simulink model "LKAS_AutoSave_20200910_1510"  (R2018b)
settings: Solver=FixedStepDiscrete  StartTime=0.0  StopTime=10.0  FixedStep=0.01  RelTol=1e-3
InitFcn:
  | tmpVer = ver('MATLAB');
  | tmpVer = str2num(tmpVer.Version);
  | % -------------------------------------------------------------------
  | %  MATLAB file generated by Simulink.saveVars on 21-Nov-2019 10:06:14
  | %  MATLAB version: 7.13.0.564 (R2011b)
  | % -------------------------------------------------------------------
  | 
  | 
  | SInt16 = Simulink.AliasType;
  | SInt16.Description = 'Num';
  | if (tmpVer > 7.11)
  | 	SInt16.DataScope = 'Auto';
  | end
  | SInt16.HeaderFile = 'Rte_Type.h';
  | SInt16.BaseType = 'int16';
  | 
  | SInt32 = Simulink.AliasType;
  | SInt32.Description = 'Num';
  | if (tmpVer > 7.11)
  | 	SInt32.DataScope = 'Auto';
  | end
  | SInt32.HeaderFile = 'Rte_Type.h';
  | SInt32.BaseType = 'int32';
  | 
  | SInt8 = Simulink.AliasType;
  | SInt8.Description = 'Num';
  | if (tmpVer > 7.11)
  | 	SInt8.DataScope = 'Auto';
  | end
  | SInt8.HeaderFile = 'Rte_Type.h';
  | SInt8.BaseType = 'int8';
  | 
  | T_A_m2_1024_1_u32 = Simulink.NumericType;
  | T_A_m2_1024_1_u32.Description = 'm2 (square meters  (m2))';
  | if (tmpVer > 7.11)
  | 	T_A_m2_1024_1_u32.DataScope = 'Auto';
  | end
  | T_A_m2_1024_1_u32.HeaderFile = 'Rte_Type.h';
  | T_A_m2_1024_1_u32.DataTypeMode = 'Fixed-point: slope and bias scaling';
  | T_A_m2_1024_1_u32.SignednessBool = false;
  | T_A_m2_1024_1_u32.WordLength = 32;
  | T_A_m2_1024_1_u32.FixedExponent = -10;
  | T_A_m2_1024_1_u32.SlopeAdjustmentFactor = 1;
  | T_A_m2_1024_1_u32.Bias = 0;
  | T_A_m2_1024_1_u32.DataTypeOverride = 'Inherit';
  | T_A_m2_1024_1_u32.IsAlias = true;
  | 
  | T_A_m2_65536_1_u16 = Simulink.NumericType;
  | T_A_m2_65536_1_u16.Description = 'm2 (square meters  (m2))';
  | if (tmpVer > 7.11)
  | 	T_A_m2_65536_1_u16.DataScope = 'Auto';
  | end
  | T_A_m2_65536_1_u16.HeaderFile = 'Rte_Type.h';
  | T_A_m2_65536_1_u16.DataTypeMode = 'Fixed-point: slope and bias scaling';
  | T_A_m2_65536_1_u16.SignednessBool = false;
  | T_A_m2_65536_1_u16.WordLength = 16;
  | T_A_m2_65536_1_u16.FixedExponent = -16;
  | T_A_m2_65536_1_u16.SlopeAdjustmentFactor = 1;
  | T_A_m2_65536_1_u16.Bias = 0;
  | T_A_m2_65536_1_u16.DataTypeOverride = 'Inherit';
  | ... (+4598 lines)
StopFcn:
  | clear  T_A_m2_1024_1_u32 T_A_m2_65536_1_u16 T_A_m2_Float32 T_A_mm2_10_1_u16 T_A_mm2_4_1_s16 T_A_mm2_Float32 T_Cnt_Num_10_1_u32 T_Cnt_Num_1_1_s16 T_Cnt_Num_1_1_s32 T_Cnt_Num_1_1_s8 T_Cnt_Num_1_1_u16 T_Cnt_Num_1_1_u32 T_Cnt_Num_1_1_u8 T_E_J_1_1_s32 T_E_J_Float32 T_E_kJ_128_1_s32 T_E_kJ_Float32 T_E_kwh_10_1_u16 T_E_kwh_Float32 T_Epl_kwhpkm_100_1_u16 T_Epl_kwhpkm_Float32 T_F_N_1_1_s16 T_F_N_Float32 T_I_A_1000_1_u16 T_I_A_1048576_1_s32 T_I_A_2048_1_s16 T_I_A_32_1_s16 T_I_A_Float32 T_I_mA_1_1_s16 T_I_mA_32768_128_s16 T_I_mA_Float32 T_J_kgpm2_128_1_u16 T_J_kgpm2_Float32 T_K_NA_1000_1_s16 T_K_NA_100_1_s16 T_K_NA_100_1_u16 T_K_NA_1024_1_s16 T_K_NA_1024_1_u16 T_K_NA_128_1_s16 T_K_NA_128_1_u16 T_K_NA_128_1_u8 T_K_NA_16777216_1_u32 T_K_NA_16_1_s16 T_K_NA_16_1_u16 T_K_NA_16_1_u8 T_K_NA_1_16_u16 T_K_NA_1_1_s16 T_K_NA_1_1_u16 T_K_NA_1_1_u8 T_K_NA_32768_1_s16 T_K_NA_32768_1_u16 T_K_NA_32_1_s8 T_K_NA_4096_1_u16 T_K_NA_4194304_1_s32 T_K_NA_4194304_1_u16 T_K_NA_65536_1_s32 T_K_NA_65536_1_u16 T_K_NA_8192_1_s16 T_K_NA_8_1_s16 T_K_NA_Float32 T_M_Nm_16_1_s16 T_M_Nm_1_1_s16 T_M_Nm_32768_1_s16 T_M_Nm_32_1_s16 T_M_Nm_4_1_s16 T_M_Nm_512_1_s16 T_M_Nm_Float32 T_P_W_1_4_s16 T_P_W_1_8_s16 T_P_W_Float32 T_P_kW_128_1_s16 T_P_kW_1_8_s16 T_P_kW_8_1_s32 T_P_kW_Float32 T_Pct_pct_1024_1_s32 T_Pct_pct_1024_1_u32 T_Pct_pct_10_1_s16 T_Pct_pct_10_1_u32 T_Pct_pct_128_100_s8 T_Pct_pct_1_1_s16 T_Pct_pct_1_4_u8 T_Pct_pct_255_100_u16 T_Pct_pct_255_100_u8 T_Pct_pct_256_1_s16 T_Pct_pct_256_1_u16 T_Pct_pct_65535_100_u16 T_Pct_pct_Float32 T_R_ohm_1024_1_s16 T_R_ohm_32_1_s16 T_R_ohm_Float32 T_TK_K_16_1_s16 T_TK_K_Float32 T_T_degC_10_400_1_u16 T_T_degC_16_1_s16 T_T_degC_1_40_1_u8 T_T_degC_2_80_1_u8 T_T_degC_Float32 T_U_V_1000_1_u16 T_U_V_10_1_u8 T_U_V_200_1_u8 T_U_V_32_1_s16 T_U_V_4096_1_s16 T_U_V_512_1_s16 T_U_V_65535_8_u16 T_U_V_8192_1_u16 T_U_V_Float32 T_U_mV_1_1_s16 T_U_mV_256_20_u16 T_U_mV_Float32 T_V_l_256_1_s16 T_V_l_4096_1_s16 T_V_l_64_1_s16 T_V_l_65535_100_u16 T_V_l_Float32 T_V_ml_128_1_s16 T_V_ml_1_1_s16 T_V_ml_32768_1_s16 T_V_ml_Float32 T_V_ul_32_1_u16 T_V_ul_Float32 T_Vpl_clpkm_512_1_u16 T_Vpl_clpkm_Float32 T_a_kphps_16_1_s16 T_a_kphps_Float32 T_a_mps2_128_1_s16 T_a_mps2_Float32 T_c_MJpkg_256_1_s16 T_c_MJpkg_Float32 T_c_kJpgpK_1024_1_s16 T_c_kJpgpK_Float32 T_c_kJpkgpK_128_1_u16 T_c_kJpkgpK_Float32 T_chrg_Ah_1_1_s16 T_chrg_Ah_1_1_u16 T_chrg_Ah_1_1_u8 T_chrg_Ah_256_1_u16 T_chrg_Ah_4194304_1_s32 T_chrg_Ah_512_1_u16 T_chrg_Ah_8_1_u16 T_chrg_Ah_Float32 T_cmp_NA_100_1_s16 T_cmp_NA_128_1_s16 T_cmp_NA_16_1_s16 T_cmp_NA_32768_1_u16 T_cmp_NA_Float32 T_d2n_rpmps2_4_1_s16 T_d2n_rpmps2_Float32 T_dPct_pctps_16_1_s16 T_dPct_pctps_256_1_s16 T_dPct_pctps_Float32 T_dT_degCps_128_1_s16 T_dT_degCps_Float32 T_dV_lph_1_1_s16 T_dV_lph_Float32 T_dV_lpm_128_1_s16 T_dV_lpm_32_1_s16 T_dV_lpm_Float32 T_dV_lps_1024_1_u16 T_dV_lps_4_1_u16 T_dV_lps_Float32 T_dV_mlps_1024_1_s16 T_dV_mlps_Float32 T_d_BitField16 T_dm_gps_128_1_s16 T_dm_gps_128_1_u16 T_dm_gps_256_1_u16 T_dm_gps_Float32 T_dm_mgps_1_1_s16 T_dm_mgps_Float32 T_dn_rpmps_1_1_s16 T_dn_rpmps_2_1_s16 T_dn_rpmps_Float32 T_dp_Paps_1_1_s16 T_dp_Paps_Float32 T_dp_kPaps_1_1_s16 T_dp_kPaps_8_1_s16 T_dp_kPaps_Float32 T_dphi_degps_128_1_s16 T_dphi_degps_8_1_s16 T_dphi_degps_Float32 T_dr_ps_256_1_s16 T_dr_ps_Float32 T_drho_mgplps_1_2_s16 T_drho_mgplps_Float32 T_e_NA_1_1_u8 T_f_Hz_1_1_u16 T_f_Hz_1_1_u32 T_f_Hz_64_1_u16 T_f_Hz_8_1_s16 T_f_Hz_Float32 T_g_BitField32 T_l_km_16_1_s16 T_l_km_1_1_u16 T_l_km_1_1_u32 T_l_km_Float32 T_l_m_1024_1_s16 T_l_m_16_1_s16 T_l_m_1_1_u32 T_l_m_Float32 T_l_mm_16_1_s16 T_l_mm_1_1_u16 T_l_mm_4096_1_s16 T_l_mm_4_1_u8 T_l_mm_64_1_s16 T_l_mm_Float32 T_m_g_1_1_s16 T_m_g_2048_1_s16 T_m_g_32_1_u16 T_m_g_Float32 T_m_kg_1024_1_s16 T_m_kg_1_1_s16 T_m_kg_1_1_u32 T_m_kg_Float32 T_m_mg_128_1_s16 T_m_mg_32_1_s16 T_m_mg_Float32 T_n_rpm_1_1_s16 T_n_rpm_1_25_u8 T_n_rpm_256_50_u16 T_n_rpm_2_25_u8 T_n_rpm_4_1_u16 T_n_rpm_Float32 T_p_MPa_64_1_s16 T_p_MPa_Float32 T_p_Pa_1_1_s16 T_p_Pa_Float32 T_p_kPa_1_10_u16 T_p_kPa_1_1_s16 T_p_kPa_1_1_u8 T_p_kPa_256_1_u16 T_p_kPa_32_1_u16 T_p_kPa_64_1_s16 T_p_kPa_Float32 T_phi_deg_100_1_s16 T_phi_deg_1024_1_s16 T_phi_deg_128_1_s16 T_phi_deg_1_1_u8 T_phi_deg_256_1_s16 T_phi_deg_2_1_s8 T_phi_deg_32_1_s16 T_phi_deg_512_6_s32 T_phi_deg_Float32 T_phi_rad_2048_1_s16 T_phi_rad_Float32 T_r_NA_1024_1_s16 T_r_NA_1024_1_u16 T_r_NA_16384_1_s16 T_r_NA_16_1_s16 T_r_NA_256_1_s8 T_r_NA_256_1_u16 T_r_NA_32768_1_u16 T_r_NA_32_1_u16 T_r_NA_4096_1_s16 T_r_NA_65535_2_u16 T_r_NA_8192_1_u16 T_r_NA_Float32 T_rho_gpl_8192_1_s16 T_rho_gpl_Float32 T_rho_kgpm3_16_1_s16 T_rho_kgpm3_Float32 T_rho_mgpl_1_1_s16 T_rho_mgpl_64_1_s16 T_rho_mgpl_Float32 T_t_hour_1_1_s16 T_t_hour_Float32 T_t_m_1_1_u16 T_t_m_Float32 T_t_ms_1_1_s16 T_t_ms_1_1_u16 T_t_ms_1_1_u32 T_t_ms_4096_1_s16 T_t_ms_64_1_s16 T_t_ms_Float32 T_t_s_1000_1_s16 T_t_s_100_1_s16 T_t_s_10_1_s16 T_t_s_10_1_u16 T_t_s_1_1_s16 T_t_s_1_1_u16 T_t_s_1_1_u32 T_t_s_Float32 T_t_us_10_1_u32 T_t_us_1_1_s16 T_t_us_1_1_u32 T_t_us_1_4_u16 T_t_us_Float32 T_v_kph_1_1_u8 T_v_kph_64_1_s16 T_v_kph_64_1_u16 T_v_kph_Float32 T_v_mps_256_1_s16 T_v_mps_Float32 T_w_radps_32_1_s16 T_w_radps_Float32 T_y_BitField8 T_y_BitFieldDiagProgress T_y_BitFieldDiagStatus T_y_NA_1_1_u8 SInt16 SInt32 SInt8 T_BOOLEAN UInt16 UInt32 UInt8 s16 s32 s8 u16 u32 u8
model workspace (MAT data in the model file):
  MCOS : class17 (value not decoded)
  MCOS : class17 (value not decoded)
  MCOS : class17 (value not decoded)
  MCOS : class17 (value not decoded)
  MCOS : class17 (value not decoded)
  MCOS : class17 (value not decoded)
  MCOS : class17 (value not decoded)
  MCOS : class17 (value not decoded)
  MCOS : class17 (value not decoded)
  MCOS : class17 (value not decoded)
  MCOS : class17 (value not decoded)
  MCOS : class17 (value not decoded)
  MCOS : class17 (value not decoded)
  MCOS : class17 (value not decoded)
  MCOS : class17 (value not decoded)
  MCOS : class17 (value not decoded)
  MCOS : class17 (value not decoded)
  MCOS : class17 (value not decoded)
  MCOS : class17 (value not decoded)
  MCOS : class17 (value not decoded)
  MCOS : class17 (value not decoded)
  MCOS : class17 (value not decoded)
  MCOS : class17 (value not decoded)
  MCOS : class17 (value not decoded)
  MCOS : class17 (value not decoded)
  MCOS : class17 (value not decoded)
  MCOS : class17 (value not decoded)
  MCOS : class17 (value not decoded)
  MCOS : class17 (value not decoded)
  MCOS : class17 (value not decoded)
  MCOS : class17 (value not decoded)
  MCOS : class17 (value not decoded)
  MCOS : class17 (value not decoded)
  MCOS : class17 (value not decoded)
  MCOS : class17 (value not decoded)
  MCOS : class17 (value not decoded)
  MCOS : class17 (value not decoded)
  MCOS : class17 (value not decoded)
  MCOS : class17 (value not decoded)
  MCOS : class17 (value not decoded)
  MCOS : class17 (value not decoded)
  MCOS : class17 (value not decoded)
  MCOS : class17 (value not decoded)
  MCOS : class17 (value not decoded)
  MCOS : class17 (value not decoded)
  MCOS : class17 (value not decoded)
  MCOS : class17 (value not decoded)
  MCOS : class17 (value not decoded)
  MCOS : class17 (value not decoded)
  MCOS : class17 (value not decoded)
  MCOS : class17 (value not decoded)
  MCOS : class17 (value not decoded)
  MCOS : class17 (value not decoded)
  MCOS : class17 (value not decoded)
  MCOS : class17 (value not decoded)
  MCOS : class17 (value not decoded)
  MCOS : class17 (value not decoded)
  MCOS : class17 (value not decoded)
  MCOS : class17 (value not decoded)
  MCOS : class17 (value not decoded)
  MCOS : class17 (value not decoded)
  MCOS : class17 (value not decoded)
  MCOS : class17 (value not decoded)
  MCOS : class17 (value not decoded)
  MCOS : class17 (value not decoded)
  MCOS : class17 (value not decoded)
  MCOS : class17 (value not decoded)
  MCOS : class17 (value not decoded)
  MCOS : class17 (value not decoded)
  MCOS : class17 (value not decoded)
  MCOS : class17 (value not decoded)
  MCOS : class17 (value not decoded)
  MCOS : class17 (value not decoded)
  MCOS : class17 (value not decoded)
  MCOS : class17 (value not decoded)
  MCOS : class17 (value not decoded)
  MCOS : class17 (value not decoded)
  MCOS : class17 (value not decoded)
  MCOS : class17 (value not decoded)
  MCOS : class17 (value not decoded)
  MCOS : class17 (value not decoded)
  MCOS : class17 (value not decoded)
  MCOS : class17 (value not decoded)
  MCOS : class17 (value not decoded)
  MCOS : class17 (value not decoded)
  MCOS : class17 (value not decoded)
  MCOS : class17 (value not decoded)
  MCOS : class17 (value not decoded)
  MCOS : class17 (value not decoded)
undefined symbols (not defined in the file): LKA_CarWidth, LKA_SampleTime, LKA_StrRatio_C, LKA_Veh2CamL_C, LKA_Veh2CamW_C, LKA_WhlBaseL_C, LL_CompSWA_C, LL_CrvtPrvwT_C, LL_DesDvt_C, LL_DvtComp_C, LL_DvtPrvwT_C, LL_DvtSpdDet_vDvtSpdMin_C, LL_HdAgExT_C, LL_HdAgPrvwT_C, LL_LAccMax_C, LL_LAccRMax_C, LL_LDW_EarliestWarnLine_C, LL_LDW_LatestWarnLine_C, LL_LDWS_SUPPRESS_HEADING, LL_LFClb_TFC_DiffCtlBalance, LL_LFClb_TFC_DiffCtrlMaxSWA, LL_LFClb_TFC_DiffCtrlRatio, LL_LFClb_TFC_facmGainLutGain1_C, LL_LFClb_TFC_facmGainLutGain2_C, LL_LFClb_TFC_facmIntegRatio, LL_LFClb_TFC_facmKlat_C, LL_LFClb_TFC_FfCtlRatio_C, LL_LFClb_TFC_phiIntegCtlMaxSWA_C, LL_LFClb_TFC_tiKlatPrvwT_C, LL_LFClb_TFC_vGainLutVehSpdLwr_C, LL_LFClb_TFC_vGainLutVehSpdUpr_C, LL_LKA_EarliestWarnLine_C, LL_LKA_LatestWarnLine_C, LL_LKAExPrcs_ExitC0Dvt, LL_LKAExPrcs_ExitC0Swt, LL_LKAExPrcs_tiExitTime1, LL_LKAExPrcs_tiExitTime2, LL_LKAExPrcs_tiExitTime3, LL_LKAS_OUT_OF_CONTROL_LAT_VEL, LL_LKAS_OUT_OF_CONTROL_TTLC, LL_LKASWASyn_M0, LL_LKASWASyn_M1, LL_LKASWASyn_M2, LL_LKASWASyn_M3K, LL_LKASWASyn_SWAaddMax, LL_LKASWASyn_T2, LL_LKASWASyn_tiTrqSwaRtTime, LL_LKASWASyn_tiTrqSwaTime, LL_LKASWASyn_TrqMax, LL_LKASWASyn_TrqSwaAddSwt, LL_LKASWASyn_TrqSwaRateDiff, LL_LSpdCompT_C, LL_lStpLngth_C, LL_MAX_DELAY_EPSSTAR_TIME, LL_MAX_DRIVER_TORQUE_DISABLE, LL_MAX_DRIVER_TORQUE_ENABLE, LL_MAX_LANE_WIDTH_DISABLE, LL_MAX_LANE_WIDTH_ENABLE, LL_MAX_LAT_ACC_DISABLE, LL_MAX_LAT_ACC_ENABLE ... (+29)
libraries: simulink x134, dspstat3 x3, simulink_extras x1
(part 5 of 19)

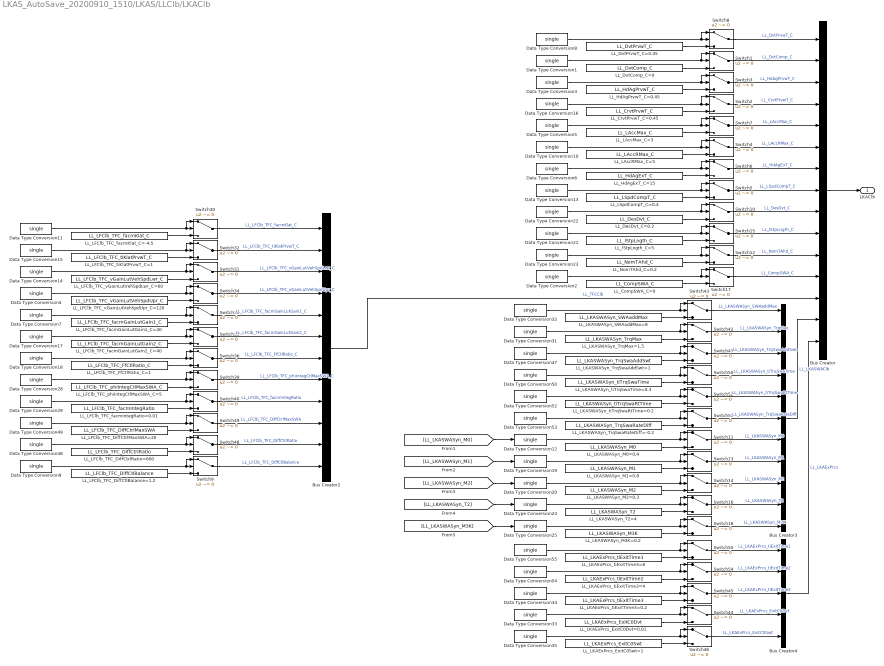
== system LKAS_AutoSave_20200910_1510/LKAS/LLClb/LKAClb ==
  Bus Creator : BusCreator  Inputs=15
  Bus Creator2 : BusCreator  Inputs=12
  Bus Creator3 : BusCreator  Inputs=11
  Bus Creator4 : BusCreator  Inputs=5
  Data Type Conversion{1..25,28..29,31..35,47..50,52..55} (40 alike) : DataTypeConversion  OutDataTypeStr=single
  LL_CompSWA_C=0 : Constant  Value=LL_CompSWA_C  OutDataTypeStr=single
  LL_CrvtPrvwT_C=0.45 : Constant  Value=LL_CrvtPrvwT_C  OutDataTypeStr=single
  LL_DesDvt_C=0.2 : Constant  Value=LL_DesDvt_C  OutDataTypeStr=single
  LL_DvtComp_C=0 : Constant  Value=LL_DvtComp_C  OutDataTypeStr=single
  LL_DvtPrvwT_C=0.45 : Constant  Value=LL_DvtPrvwT_C  OutDataTypeStr=single
  LL_HdAgExT_C=15 : Constant  Value=LL_HdAgExT_C  OutDataTypeStr=single
  LL_HdAgPrvwT_C=0.45 : Constant  Value=LL_HdAgPrvwT_C  OutDataTypeStr=single
  LL_LAccMax_C=3 : Constant  Value=LL_LAccMax_C  OutDataTypeStr=single
  LL_LAccRMax_C=5 : Constant  Value=LL_LAccRMax_C  OutDataTypeStr=single
  LL_LFClb_TFC_DiffCtlBalance=1.2 : Constant  Value=LL_LFClb_TFC_DiffCtlBalance  OutDataTypeStr=single
  LL_LFClb_TFC_DiffCtrlMaxSWA=20 : Constant  Value=LL_LFClb_TFC_DiffCtrlMaxSWA  OutDataTypeStr=single
  LL_LFClb_TFC_DiffCtrlRatio=600 : Constant  Value=LL_LFClb_TFC_DiffCtrlRatio  OutDataTypeStr=single
  LL_LFClb_TFC_FfCtlRatio_C=1 : Constant  Value=LL_LFClb_TFC_FfCtlRatio_C  OutDataTypeStr=single
  LL_LFClb_TFC_facmGainLutGain1_C=40 : Constant  Value=LL_LFClb_TFC_facmGainLutGain1_C  OutDataTypeStr=single
  LL_LFClb_TFC_facmGainLutGain2_C=40 : Constant  Value=LL_LFClb_TFC_facmGainLutGain2_C  OutDataTypeStr=single
  LL_LFClb_TFC_facmIntegRatio=0.01 : Constant  Value=LL_LFClb_TFC_facmIntegRatio  OutDataTypeStr=single
  LL_LFClb_TFC_facmKlat_C=-4.5 : Constant  Value=LL_LFClb_TFC_facmKlat_C  OutDataTypeStr=single
  LL_LFClb_TFC_phiIntegCtlMaxSWA_C=5 : Constant  Value=LL_LFClb_TFC_phiIntegCtlMaxSWA_C  OutDataTypeStr=single
  LL_LFClb_TFC_tiKlatPrvwT_C=1 : Constant  Value=LL_LFClb_TFC_tiKlatPrvwT_C  OutDataTypeStr=single
  LL_LFClb_TFC_vGainLutVehSpdLwr_C=60 : Constant  Value=LL_LFClb_TFC_vGainLutVehSpdLwr_C  OutDataTypeStr=single
  LL_LFClb_TFC_vGainLutVehSpdUpr_C=120 : Constant  Value=LL_LFClb_TFC_vGainLutVehSpdUpr_C  OutDataTypeStr=single
  LL_LKAExPrcs_ExitC0Dvt=0.01 : Constant  Value=LL_LKAExPrcs_ExitC0Dvt  OutDataTypeStr=single
  LL_LKAExPrcs_ExitC0Swt=1 : Constant  Value=LL_LKAExPrcs_ExitC0Swt  OutDataTypeStr=single
  LL_LKAExPrcs_tiExitTime3=0.2 : Constant  Value=LL_LKAExPrcs_tiExitTime3  OutDataTypeStr=single
  LL_LKAExPrcs_tiExitTime3=4 : Constant  Value=LL_LKAExPrcs_tiExitTime2  OutDataTypeStr=single
  LL_LKAExPrcs_tiExitTime3=8 : Constant  Value=LL_LKAExPrcs_tiExitTime1  OutDataTypeStr=single
  LL_LKASWASyn_M0=0.4 : Constant  Value=LL_LKASWASyn_M0  OutDataTypeStr=single
  LL_LKASWASyn_M1=0.8 : Constant  Value=LL_LKASWASyn_M1  OutDataTypeStr=single
  LL_LKASWASyn_M2=0.3 : Constant  Value=LL_LKASWASyn_M2  OutDataTypeStr=single
  LL_LKASWASyn_M3K=0.2 : Constant  Value=LL_LKASWASyn_M3K  OutDataTypeStr=single
  LL_LKASWASyn_SWAaddMax=8 : Constant  Value=LL_LKASWASyn_SWAaddMax  OutDataTypeStr=single
  LL_LKASWASyn_T2=4 : Constant  Value=LL_LKASWASyn_T2  OutDataTypeStr=single
  LL_LKASWASyn_TrqMax=1.5 : Constant  Value=LL_LKASWASyn_TrqMax  OutDataTypeStr=single
  LL_LKASWASyn_TrqSwaAddSwt=1 : Constant  Value=LL_LKASWASyn_TrqSwaAddSwt  OutDataTypeStr=single
  LL_LKASWASyn_TrqSwaRateDiff=-0.2 : Constant  Value=LL_LKASWASyn_TrqSwaRateDiff  OutDataTypeStr=single
  LL_LKASWASyn_tiTrqSwaRtTime=0.2 : Constant  Value=LL_LKASWASyn_tiTrqSwaRtTime  OutDataTypeStr=single
  LL_LKASWASyn_tiTrqSwaTime=0.3 : Constant  Value=LL_LKASWASyn_tiTrqSwaTime  OutDataTypeStr=single
  LL_LSpdCompT_C=0.4 : Constant  Value=LL_LSpdCompT_C  OutDataTypeStr=single
  LL_NomTAhd_C=0.2 : Constant  Value=LL_NomTAhd_C  OutDataTypeStr=single
  LL_lStpLngth_C=5 : Constant  Value=LL_lStpLngth_C  OutDataTypeStr=single
  Switch{1..18,30..36,39..40,42..50,52..55} (40 alike) : Switch  Criteria=u2 ~= 0  OutDataTypeStr=single
  LKAClb : Outport
  wires:
  [LL_LKASWASyn_M3K] -> Data Type Conversion25/1
  Switch18/1 -> Bus Creator3/11  "LL_LKASWASyn_M3K"
  LL_LKASWASyn_M3K=0.2/1 -> Switch18/3
  Data Type Conversion25/1 -> Switch18/1, Switch18/2
  [LL_LKASWASyn_M0] -> Data Type Conversion12/1
  Switch11/1 -> Bus Creator3/7  "LL_LKASWASyn_M0"
  LL_LKASWASyn_M0=0.4/1 -> Switch11/3
  Data Type Conversion12/1 -> Switch11/1, Switch11/2
  Data Type Conversion19/1 -> Switch13/2, Switch13/1
  LL_LKASWASyn_M1=0.8/1 -> Switch13/3
  Switch13/1 -> Bus Creator3/8  "LL_LKASWASyn_M1"
  [LL_LKASWASyn_M1] -> Data Type Conversion19/1
  [LL_LKASWASyn_M2] -> Data Type Conversion20/1
  Switch14/1 -> Bus Creator3/9  "LL_LKASWASyn_M2"
  LL_LKASWASyn_M2=0.3/1 -> Switch14/3
  Data Type Conversion20/1 -> Switch14/1, Switch14/2
  Data Type Conversion24/1 -> Switch16/2, Switch16/1
  LL_LKASWASyn_T2=4/1 -> Switch16/3
  Switch16/1 -> Bus Creator3/10  "LL_LKASWASyn_T2"
  [LL_LKASWASyn_T2] -> Data Type Conversion24/1
  Data Type Conversion9/1 -> Switch9/2, Switch9/1
  LL_LFClb_TFC_DiffCtlBalance=1.2/1 -> Switch9/3
  Switch9/1 -> Bus Creator2/12  "LL_LFClb_TFC_DiffCtlBalance"
  LL_LKAExPrcs_tiExitTime3=8/1 -> Switch55/3
  Data Type Conversion55/1 -> Switch55/1, Switch55/2
  Switch55/1 -> Bus Creator4/1  "LL_LKAExPrcs_tiExitTime1"
  Switch54/1 -> Bus Creator4/2  "LL_LKAExPrcs_tiExitTime2"
  Data Type Conversion54/1 -> Switch54/2, Switch54/1
  LL_LKAExPrcs_tiExitTime3=4/1 -> Switch54/3
  Switch53/1 -> Bus Creator3/6  "LL_LKASWASyn_TrqSwaRateDiff"
  LL_LKASWASyn_TrqSwaRateDiff=-0.2/1 -> Switch53/3
  Data Type Conversion53/1 -> Switch53/1, Switch53/2
  Data Type Conversion52/1 -> Switch52/2, Switch52/1
  LL_LKASWASyn_tiTrqSwaRtTime=0.2/1 -> Switch52/3
  Switch52/1 -> Bus Creator3/5  "LL_LKASWASyn_tiTrqSwaRtTime"
  Switch50/1 -> Bus Creator3/4  "LL_LKASWASyn_tiTrqSwaTime"
  LL_LKASWASyn_tiTrqSwaTime=0.3/1 -> Switch50/3
  Data Type Conversion50/1 -> Switch50/1, Switch50/2
  Data Type Conversion49/1 -> Switch49/2, Switch49/1
  LL_LFClb_TFC_DiffCtrlMaxSWA=20/1 -> Switch49/3
  Switch49/1 -> Bus Creator2/10  "LL_LFClb_TFC_DiffCtrlMaxSWA"
  Switch48/1 -> Bus Creator2/11  "LL_LFClb_TFC_DiffCtrlRatio"
  LL_LFClb_TFC_DiffCtrlRatio=600/1 -> Switch48/3
  Data Type Conversion48/1 -> Switch48/1, Switch48/2
  Data Type Conversion47/1 -> Switch47/2, Switch47/1
  LL_LKASWASyn_TrqSwaAddSwt=1/1 -> Switch47/3
  Switch47/1 -> Bus Creator3/3  "LL_LKASWASyn_TrqSwaAddSwt"
  Switch46/1 -> Bus Creator4/5  "LL_LKAExPrcs_ExitC0Swt"
  LL_LKAExPrcs_ExitC0Swt=1/1 -> Switch46/3
  Data Type Conversion35/1 -> Switch46/1, Switch46/2
  Bus Creator4/1 -> Bus Creator/15  "LL_LKAExPrcs"
  Data Type Conversion33/1 -> Switch44/2, Switch44/1
  LL_LKAExPrcs_ExitC0Dvt=0.01/1 -> Switch44/3
  LL_LKAExPrcs_tiExitTime3=0.2/1 -> Switch45/3
  Data Type Conversion34/1 -> Switch45/1, Switch45/2
  Switch45/1 -> Bus Creator4/3  "LL_LKAExPrcs_tiExitTime3"
  Switch44/1 -> Bus Creator4/4  "LL_LKAExPrcs_ExitC0Dvt"
  Bus Creator3/1 -> Bus Creator/14  "LL_LKASWAClb"
  Switch42/1 -> Bus Creator3/2  "LL_LKASWASyn_TrqMax"
  Switch43/1 -> Bus Creator3/1  "LL_LKASWASyn_SWAaddMax"
  Data Type Conversion32/1 -> Switch43/2, Switch43/1
  LL_LKASWASyn_SWAaddMax=8/1 -> Switch43/3
  LL_LKASWASyn_TrqMax=1.5/1 -> Switch42/3
  Data Type Conversion31/1 -> Switch42/1, Switch42/2
  Data Type Conversion29/1 -> Switch40/2, Switch40/1
  LL_LFClb_TFC_facmIntegRatio=0.01/1 -> Switch40/3
  Data Type Conversion28/1 -> Switch39/2, Switch39/1
  LL_LFClb_TFC_phiIntegCtlMaxSWA_C=5/1 -> Switch39/3
  Switch39/1 -> Bus Creator2/8  "LL_LFClb_TFC_phiIntegCtlMaxSWA_C"
  Switch40/1 -> Bus Creator2/9  "LL_LFClb_TFC_facmIntegRatio"
  Switch36/1 -> Bus Creator2/7  "LL_LFClb_TFC_FfCtlRatio_C"
  Data Type Conversion18/1 -> Switch36/2, Switch36/1
  LL_LFClb_TFC_FfCtlRatio_C=1/1 -> Switch36/3
  LL_LFClb_TFC_facmKlat_C=-4.5/1 -> Switch30/3
  LL_LFClb_TFC_vGainLutVehSpdUpr_C=120/1 -> Switch34/3
  Data Type Conversion14/1 -> Switch31/1, Switch31/2
  LL_LFClb_TFC_facmGainLutGain2_C=40/1 -> Switch35/3
  Data Type Conversion17/1 -> Switch35/1, Switch35/2
  Data Type Conversion15/1 -> Switch32/1, Switch32/2
  Data Type Conversion4/1 -> Switch34/1, Switch34/2
  Data Type Conversion7/1 -> Switch33/1, Switch33/2
  Data Type Conversion11/1 -> Switch30/1, Switch30/2
  LL_LFClb_TFC_tiKlatPrvwT_C=1/1 -> Switch32/3
  LL_LFClb_TFC_vGainLutVehSpdLwr_C=60/1 -> Switch31/3
  LL_LFClb_TFC_facmGainLutGain1_C=40/1 -> Switch33/3
  Switch32/1 -> Bus Creator2/2  "LL_LFClb_TFC_tiKlatPrvwT_C"
  Switch33/1 -> Bus Creator2/5  "LL_LFClb_TFC_facmGainLutGain1_C"
  Switch34/1 -> Bus Creator2/4  "LL_LFClb_TFC_vGainLutVehSpdUpr_C"
  Switch31/1 -> Bus Creator2/3  "LL_LFClb_TFC_vGainLutVehSpdLwr_C"
  Switch30/1 -> Bus Creator2/1  "LL_LFClb_TFC_facmKlat_C"
  Switch35/1 -> Bus Creator2/6  "LL_LFClb_TFC_facmGainLutGain2_C"
  Bus Creator2/1 -> Bus Creator/13  "LL_TFCClb"
  LL_CompSWA_C=0/1 -> Switch17/3
  LL_NomTAhd_C=0.2/1 -> Switch12/3
  LL_lStpLngth_C=5/1 -> Switch15/3
  LL_DesDvt_C=0.2/1 -> Switch10/3
  Data Type Conversion2/1 -> Switch17/1, Switch17/2
  Data Type Conversion22/1 -> Switch10/1, Switch10/2
  Data Type Conversion23/1 -> Switch12/1, Switch12/2
  Data Type Conversion21/1 -> Switch15/1, Switch15/2
  LL_LAccMax_C=3/1 -> Switch7/3
  Data Type Conversion5/1 -> Switch7/1, Switch7/2
  Data Type Conversion10/1 -> Switch4/2, Switch4/1
  LL_LAccRMax_C=5/1 -> Switch4/3
  LL_LSpdCompT_C=0.4/1 -> Switch5/3
  Data Type Conversion13/1 -> Switch5/1, Switch5/2
  Data Type Conversion6/1 -> Switch6/1, Switch6/2
  LL_HdAgExT_C=15/1 -> Switch6/3
  LL_HdAgPrvwT_C=0.45/1 -> Switch3/3
  Data Type Conversion3/1 -> Switch3/1, Switch3/2
  Data Type Conversion16/1 -> Switch2/1, Switch2/2
  LL_CrvtPrvwT_C=0.45/1 -> Switch2/3
  LL_DvtComp_C=0/1 -> Switch1/3
  Data Type Conversion1/1 -> Switch1/1, Switch1/2
  Data Type Conversion8/1 -> Switch8/2, Switch8/1
  LL_DvtPrvwT_C=0.45/1 -> Switch8/3
  Switch12/1 -> Bus Creator/11  "LL_NomTAhd_C"
  Switch10/1 -> Bus Creator/9  "LL_DesDvt_C"
  Switch15/1 -> Bus Creator/10  "LL_lStpLngth_C"
  Switch2/1 -> Bus Creator/4  "LL_CrvtPrvwT_C"
  Switch5/1 -> Bus Creator/8  "LL_LSpdCompT_C"
  Switch4/1 -> Bus Creator/6  "LL_LAccRMax_C"
  Switch7/1 -> Bus Creator/5  "LL_LAccMax_C"
  Switch6/1 -> Bus Creator/7  "LL_HdAgExT_C"
  Switch17/1 -> Bus Creator/12  "LL_CompSWA_C"
  Switch3/1 -> Bus Creator/3  "LL_HdAgPrvwT_C"
  Switch1/1 -> Bus Creator/2  "LL_DvtComp_C"
  Switch8/1 -> Bus Creator/1  "LL_DvtPrvwT_C"
  Bus Creator/1 -> LKAClb/1

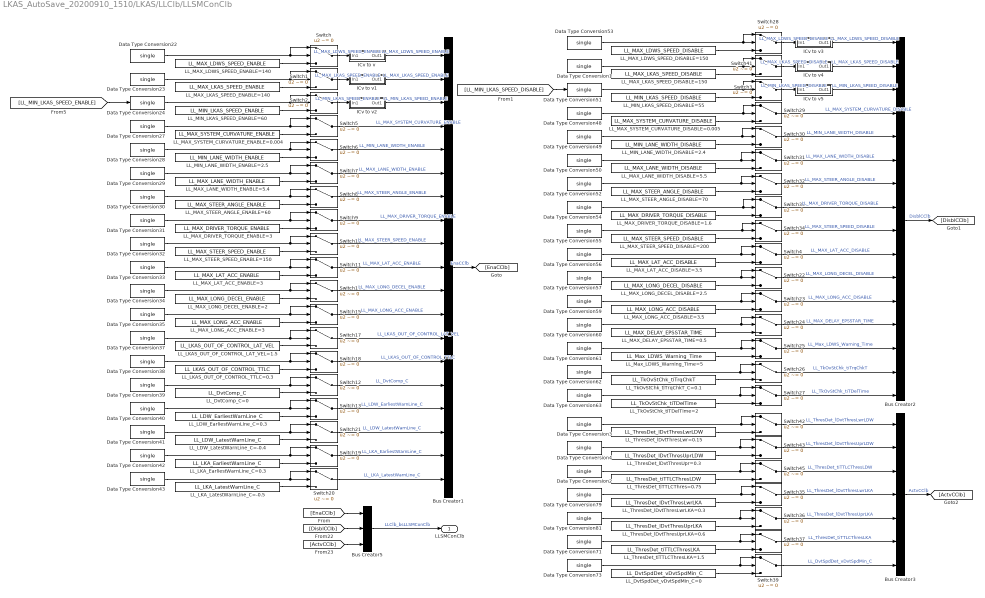
== system LKAS_AutoSave_20200910_1510/LKAS/LLClb/LLSMConClb ==
  Bus Creator1 : BusCreator  Inputs=19
  Bus Creator2 : BusCreator  Inputs=16
  Bus Creator3 : BusCreator  Inputs=7
  Bus Creator5 : BusCreator  Inputs=3
  Data Type Conversion{1..4,22..24,27..35,37..43,48..57,59..63,71,73,79,81} (42 alike) : DataTypeConversion  OutDataTypeStr=single
  ICv to v : Subsystem
  ICv to v1 : Subsystem
  ICv to v2 : Subsystem
  ICv to v3 : Subsystem
  ICv to v4 : Subsystem
  ICv to v5 : Subsystem
  LL_DvtComp_C=0 : Constant  Value=LL_DvtComp_C  OutDataTypeStr=single
  LL_DvtSpdDet_vDvtSpdMin_C=0 : Constant  Value=LL_DvtSpdDet_vDvtSpdMin_C  OutDataTypeStr=single
  LL_LDW_EarliestWarnLine_C=0.3 : Constant  Value=LL_LDW_EarliestWarnLine_C  OutDataTypeStr=single
  LL_LDW_LatestWarnLine_C=-0.4 : Constant  Value=LL_LDW_LatestWarnLine_C  OutDataTypeStr=single
  LL_LKAS_OUT_OF_CONTROL_LAT_VEL=1.5 : Constant  Value=LL_LKAS_OUT_OF_CONTROL_LAT_VEL  OutDataTypeStr=single
  LL_LKAS_OUT_OF_CONTROL_TTLC=0.3 : Constant  Value=LL_LKAS_OUT_OF_CONTROL_TTLC  OutDataTypeStr=single
  LL_LKA_EarliestWarnLine_C=0.3 : Constant  Value=LL_LKA_EarliestWarnLine_C  OutDataTypeStr=single
  LL_LKA_LatestWarnLine_C=-0.5 : Constant  Value=LL_LKA_LatestWarnLine_C  OutDataTypeStr=single
  LL_MAX_DELAY_EPSSTAR_TIME=0.5 : Constant  Value=LL_MAX_DELAY_EPSSTAR_TIME  OutDataTypeStr=single
  LL_MAX_DRIVER_TORQUE_DISABLE=1.6 : Constant  Value=LL_MAX_DRIVER_TORQUE_DISABLE  OutDataTypeStr=single
  LL_MAX_DRIVER_TORQUE_ENABLE=3 : Constant  Value=LL_MAX_DRIVER_TORQUE_ENABLE  OutDataTypeStr=single
  LL_MAX_LANE_WIDTH_DISABLE=5.5 : Constant  Value=LL_MAX_LANE_WIDTH_DISABLE  OutDataTypeStr=single
  LL_MAX_LANE_WIDTH_ENABLE=5.4 : Constant  Value=LL_MAX_LANE_WIDTH_ENABLE  OutDataTypeStr=single
  LL_MAX_LAT_ACC_DISABLE=3.5 : Constant  Value=LL_MAX_LAT_ACC_DISABLE  OutDataTypeStr=single
  LL_MAX_LAT_ACC_ENABLE=3 : Constant  Value=LL_MAX_LAT_ACC_ENABLE  OutDataTypeStr=single
  LL_MAX_LDWS_SPEED_DISABLE=150 : Constant  Value=LL_MAX_LDWS_SPEED_DISABLE  OutDataTypeStr=single
  LL_MAX_LDWS_SPEED_ENABLE=140 : Constant  Value=LL_MAX_LDWS_SPEED_ENABLE  OutDataTypeStr=single
  LL_MAX_LKAS_SPEED_DISABLE=150 : Constant  Value=LL_MAX_LKAS_SPEED_DISABLE  OutDataTypeStr=single
  LL_MAX_LKAS_SPEED_ENABLE=140 : Constant  Value=LL_MAX_LKAS_SPEED_ENABLE  OutDataTypeStr=single
  LL_MAX_LONG_ACC_DISABLE=3.5 : Constant  Value=LL_MAX_LONG_ACC_DISABLE  OutDataTypeStr=single
  LL_MAX_LONG_ACC_ENABLE=3 : Constant  Value=LL_MAX_LONG_ACC_ENABLE  OutDataTypeStr=single
  LL_MAX_LONG_DECEL_DISABLE=2.5 : Constant  Value=LL_MAX_LONG_DECEL_DISABLE  OutDataTypeStr=single
  LL_MAX_LONG_DECEL_ENABLE=2 : Constant  Value=LL_MAX_LONG_DECEL_ENABLE  OutDataTypeStr=single
  LL_MAX_STEER_ANGLE_DISABLE=70 : Constant  Value=LL_MAX_STEER_ANGLE_DISABLE  OutDataTypeStr=single
  LL_MAX_STEER_ANGLE_ENABLE=60 : Constant  Value=LL_MAX_STEER_ANGLE_ENABLE  OutDataTypeStr=single
  LL_MAX_STEER_SPEED_DISABLE=200 : Constant  Value=LL_MAX_STEER_SPEED_DISABLE  OutDataTypeStr=single
  LL_MAX_STEER_SPEED_ENABLE=150 : Constant  Value=LL_MAX_STEER_SPEED_ENABLE  OutDataTypeStr=single
  LL_MAX_SYSTEM_CURVATURE_DISABLE=0.005 : Constant  Value=LL_MAX_SYSTEM_CURVATURE_DISABLE  OutDataTypeStr=single
  LL_MAX_SYSTEM_CURVATURE_ENABLE=0.004 : Constant  Value=LL_MAX_SYSTEM_CURVATURE_ENABLE  OutDataTypeStr=single
  LL_MIN_LANE_WIDTH_DISABLE=2.4 : Constant  Value=LL_MIN_LANE_WIDTH_DISABLE  OutDataTypeStr=single
  LL_MIN_LANE_WIDTH_ENABLE=2.5 : Constant  Value=LL_MIN_LANE_WIDTH_ENABLE  OutDataTypeStr=single
  LL_MIN_LKAS_SPEED_DISABLE=55 : Constant  Value=LL_MIN_LKAS_SPEED_DISABLE  OutDataTypeStr=single
  LL_MIN_LKAS_SPEED_ENABLE=60 : Constant  Value=LL_MIN_LKAS_SPEED_ENABLE  OutDataTypeStr=single
  LL_Max_LDWS_Warning_Time=5 : Constant  Value=LL_Max_LDWS_Warning_Time  OutDataTypeStr=single
  LL_ThresDet_lDvtThresLwr=0.15 : Constant  Value=LL_ThresDet_lDvtThresLwrLDW  OutDataTypeStr=single
  LL_ThresDet_lDvtThresLwrLKA=0.3 : Constant  Value=LL_ThresDet_lDvtThresLwrLKA  OutDataTypeStr=single
  LL_ThresDet_lDvtThresUpr=0.3 : Constant  Value=LL_ThresDet_lDvtThresUprLDW  OutDataTypeStr=single
  LL_ThresDet_lDvtThresUprLKA=0.6 : Constant  Value=LL_ThresDet_lDvtThresUprLKA  OutDataTypeStr=single
  LL_ThresDet_tiTTLCThres=0.75 : Constant  Value=LL_ThresDet_tiTTLCThresLDW  OutDataTypeStr=single
  LL_ThresDet_tiTTLCThresLKA=1.5 : Constant  Value=LL_ThresDet_tiTTLCThresLKA  OutDataTypeStr=single
  LL_TkOvStChk_tiTDelTime=2 : Constant  Value=LL_TkOvStChk_tiTDelTime  OutDataTypeStr=single
  LL_TkOvStChk_tiTrqChkT_C=0.1 : Constant  Value=LL_TkOvStChk_tiTrqChkT  OutDataTypeStr=single
  Switch{,1..15,17..37,39,41..43,45} (42 alike) : Switch  Criteria=u2 ~= 0  OutDataTypeStr=single
  LLSMConClb : Outport
  wires:
  [LL_MIN_LKAS_SPEED_DISABLE] -> Data Type Conversion51/1
  [LL_MIN_LKAS_SPEED_ENABLE] -> Data Type Conversion24/1
  Switch3/1 -> ICv to v5/1(In1)  "LL_MIN_LKAS_SPEED_DISABLE"
  Switch41/1 -> ICv to v4/1(In1)  "LL_MAX_LKAS_SPEED_DISABLE"
  ICv to v3/1(Out1) -> Bus Creator2/1  "LL_MAX_LDWS_SPEED_DISABLE"
  Switch28/1 -> ICv to v3/1(In1)  "LL_MAX_LDWS_SPEED_DISABLE"
  Switch2/1 -> ICv to v2/1(In1)  "LL_MIN_LKAS_SPEED_ENABLE"
  Switch1/1 -> ICv to v1/1(In1)  "LL_MAX_LKAS_SPEED_ENABLE"
  Switch/1 -> ICv to v/1(In1)  "LL_MAX_LDWS_SPEED_ENABLE"
  Data Type Conversion4/1 -> Switch43/2, Switch43/1
  LL_ThresDet_tiTTLCThres=0.75/1 -> Switch45/3
  Data Type Conversion2/1 -> Switch45/2, Switch45/1
  LL_ThresDet_lDvtThresLwr=0.15/1 -> Switch42/3
  Data Type Conversion3/1 -> Switch42/1, Switch42/2
  LL_ThresDet_lDvtThresUpr=0.3/1 -> Switch43/3
  Switch45/1 -> Bus Creator3/3  "LL_ThresDet_tiTTLCThresLDW"
  Switch42/1 -> Bus Creator3/1  "LL_ThresDet_lDvtThresLwrLDW"
  Switch43/1 -> Bus Creator3/2  "LL_ThresDet_lDvtThresUprLDW"
  LL_MAX_LKAS_SPEED_DISABLE=150/1 -> Switch41/3
  Data Type Conversion1/1 -> Switch41/1, Switch41/2
  ICv to v4/1(Out1) -> Bus Creator2/2  "LL_MAX_LKAS_SPEED_DISABLE"
  Bus Creator5/1 -> LLSMConClb/1  "LLClb_bsLLSMConClb"
  [ActvCClb] -> Bus Creator5/3
  [DisblCClb] -> Bus Creator5/2
  [EnaCClb] -> Bus Creator5/1
  Bus Creator3/1 -> [ActvCClb]  "ActvCClb"
  Bus Creator1/1 -> [EnaCClb]  "EnaCClb"
  Data Type Conversion73/1 -> Switch39/2, Switch39/1
  Switch36/1 -> Bus Creator3/5  "LL_ThresDet_lDvtThresUprLKA"
  Switch35/1 -> Bus Creator3/4  "LL_ThresDet_lDvtThresLwrLKA"
  Switch37/1 -> Bus Creator3/6  "LL_ThresDet_tiTTLCThresLKA"
  Switch39/1 -> Bus Creator3/7  "LL_DvtSpdDet_vDvtSpdMin_C"
  LL_ThresDet_lDvtThresUprLKA=0.6/1 -> Switch36/3
  Data Type Conversion79/1 -> Switch35/2, Switch35/1
  LL_ThresDet_lDvtThresLwrLKA=0.3/1 -> Switch35/3
  Data Type Conversion71/1 -> Switch37/1, Switch37/2
  LL_DvtSpdDet_vDvtSpdMin_C=0/1 -> Switch39/3
  LL_ThresDet_tiTTLCThresLKA=1.5/1 -> Switch37/3
  Data Type Conversion81/1 -> Switch36/1, Switch36/2
  Bus Creator2/1 -> [DisblCClb]  "DisblCClb"
  Switch27/1 -> Bus Creator2/16  "LL_TkOvStChk_tiTDelTime"
  LL_TkOvStChk_tiTDelTime=2/1 -> Switch27/3
  ICv to v5/1(Out1) -> Bus Creator2/3  "LL_MIN_LKAS_SPEED_DISABLE"
  LL_MAX_STEER_ANGLE_DISABLE=70/1 -> Switch32/3
  Data Type Conversion56/1 -> Switch4/2, Switch4/1
  Switch31/1 -> Bus Creator2/6  "LL_MAX_LANE_WIDTH_DISABLE"
  Switch34/1 -> Bus Creator2/9  "LL_MAX_STEER_SPEED_DISABLE"
  Switch32/1 -> Bus Creator2/7  "LL_MAX_STEER_ANGLE_DISABLE"
  Switch24/1 -> Bus Creator2/13  "LL_MAX_DELAY_EPSSTAR_TIME"
  Switch22/1 -> Bus Creator2/11  "LL_MAX_LONG_DECEL_DISABLE"
  LL_MAX_LONG_ACC_DISABLE=3.5/1 -> Switch23/3
  LL_MAX_STEER_SPEED_DISABLE=200/1 -> Switch34/3
  LL_Max_LDWS_Warning_Time=5/1 -> Switch25/3
  LL_MIN_LANE_WIDTH_DISABLE=2.4/1 -> Switch30/3
  Switch33/1 -> Bus Creator2/8  "LL_MAX_DRIVER_TORQUE_DISABLE"
  Data Type Conversion55/1 -> Switch34/1, Switch34/2
  LL_MAX_LAT_ACC_DISABLE=3.5/1 -> Switch4/3
  Data Type Conversion51/1 -> Switch3/2, Switch3/1
  Data Type Conversion50/1 -> Switch31/1, Switch31/2
  Switch4/1 -> Bus Creator2/10  "LL_MAX_LAT_ACC_DISABLE"
  LL_MAX_LDWS_SPEED_DISABLE=150/1 -> Switch28/3
  LL_TkOvStChk_tiTrqChkT_C=0.1/1 -> Switch26/3
  LL_MAX_LANE_WIDTH_DISABLE=5.5/1 -> Switch31/3
  LL_MAX_DRIVER_TORQUE_DISABLE=1.6/1 -> Switch33/3
  Data Type Conversion53/1 -> Switch28/1, Switch28/2
  LL_MAX_DELAY_EPSSTAR_TIME=0.5/1 -> Switch24/3
  Switch23/1 -> Bus Creator2/12  "LL_MAX_LONG_ACC_DISABLE"
  LL_MAX_SYSTEM_CURVATURE_DISABLE=0.005/1 -> Switch29/3
  Data Type Conversion48/1 -> Switch29/1, Switch29/2
  Switch29/1 -> Bus Creator2/4  "LL_MAX_SYSTEM_CURVATURE_DISABLE"
  Data Type Conversion57/1 -> Switch22/2, Switch22/1
  Switch25/1 -> Bus Creator2/14  "LL_Max_LDWS_Warning_Time"
  LL_MAX_LONG_DECEL_DISABLE=2.5/1 -> Switch22/3
  Data Type Conversion62/1 -> Switch26/1, Switch26/2
  Switch30/1 -> Bus Creator2/5  "LL_MIN_LANE_WIDTH_DISABLE"
  Data Type Conversion49/1 -> Switch30/1, Switch30/2
  Data Type Conversion59/1 -> Switch23/1, Switch23/2
  Data Type Conversion60/1 -> Switch24/1, Switch24/2
  LL_MIN_LKAS_SPEED_DISABLE=55/1 -> Switch3/3
  Switch26/1 -> Bus Creator2/15  "LL_TkOvStChk_tiTrqChkT"
  Data Type Conversion61/1 -> Switch25/1, Switch25/2
  Data Type Conversion52/1 -> Switch32/1, Switch32/2
  Data Type Conversion63/1 -> Switch27/1, Switch27/2
  Data Type Conversion54/1 -> Switch33/1, Switch33/2
  Switch11/1 -> Bus Creator1/10  "LL_MAX_LAT_ACC_ENABLE"
  LL_MAX_LKAS_SPEED_ENABLE=140/1 -> Switch1/3
  ICv to v1/1(Out1) -> Bus Creator1/2  "LL_MAX_LKAS_SPEED_ENABLE"
  LL_LDW_EarliestWarnLine_C=0.3/1 -> Switch13/3
  Data Type Conversion41/1 -> Switch21/1, Switch21/2
  Switch8/1 -> Bus Creator1/7  "LL_MAX_STEER_ANGLE_ENABLE"
  Switch5/1 -> Bus Creator1/4  "LL_MAX_SYSTEM_CURVATURE_ENABLE"
  LL_MAX_SYSTEM_CURVATURE_ENABLE=0.004/1 -> Switch5/3
  LL_MAX_STEER_SPEED_ENABLE=150/1 -> Switch10/3
  Switch9/1 -> Bus Creator1/8  "LL_MAX_DRIVER_TORQUE_ENABLE"
  Switch13/1 -> Bus Creator1/16  "LL_LDW_EarliestWarnLine_C"
  Switch14/1 -> Bus Creator1/11  "LL_MAX_LONG_DECEL_ENABLE"
  Switch20/1 -> Bus Creator1/19  "LL_LKA_LatestWarnLine_C"
  ICv to v/1(Out1) -> Bus Creator1/1  "LL_MAX_LDWS_SPEED_ENABLE"
  Switch21/1 -> Bus Creator1/17  "LL_LDW_LatestWarnLine_C"
  Switch18/1 -> Bus Creator1/14  "LL_LKAS_OUT_OF_CONTROL_TTLC"
  Switch15/1 -> Bus Creator1/12  "LL_MAX_LONG_ACC_ENABLE"
  LL_LKA_EarliestWarnLine_C=0.3/1 -> Switch19/3
  Data Type Conversion34/1 -> Switch14/1, Switch14/2
  Switch7/1 -> Bus Creator1/6  "LL_MAX_LANE_WIDTH_ENABLE"
  Data Type Conversion33/1 -> Switch11/1, Switch11/2
  Data Type Conversion37/1 -> Switch17/1, Switch17/2
  Data Type Conversion32/1 -> Switch10/1, Switch10/2
  LL_LKAS_OUT_OF_CONTROL_TTLC=0.3/1 -> Switch18/3
  Switch19/1 -> Bus Creator1/18  "LL_LKA_EarliestWarnLine_C"
  LL_DvtComp_C=0/1 -> Switch12/3
  Data Type Conversion35/1 -> Switch15/1, Switch15/2
  LL_MAX_DRIVER_TORQUE_ENABLE=3/1 -> Switch9/3
  LL_MAX_LONG_ACC_ENABLE=3/1 -> Switch15/3
  Data Type Conversion29/1 -> Switch7/1, Switch7/2
  LL_LDW_LatestWarnLine_C=-0.4/1 -> Switch21/3
  Switch12/1 -> Bus Creator1/15  "LL_DvtComp_C"
  LL_MAX_LDWS_SPEED_ENABLE=140/1 -> Switch/3
  LL_MAX_LAT_ACC_ENABLE=3/1 -> Switch11/3
  Data Type Conversion24/1 -> Switch2/1, Switch2/2
  Data Type Conversion22/1 -> Switch/1, Switch/2
  LL_MIN_LKAS_SPEED_ENABLE=60/1 -> Switch2/3
  Data Type Conversion23/1 -> Switch1/1, Switch1/2
  LL_LKAS_OUT_OF_CONTROL_LAT_VEL=1.5/1 -> Switch17/3
  Data Type Conversion28/1 -> Switch6/1, Switch6/2
  Data Type Conversion31/1 -> Switch9/1, Switch9/2
  Data Type Conversion27/1 -> Switch5/1, Switch5/2
  Data Type Conversion30/1 -> Switch8/1, Switch8/2
  LL_MAX_LONG_DECEL_ENABLE=2/1 -> Switch14/3
  Switch17/1 -> Bus Creator1/13  "LL_LKAS_OUT_OF_CONTROL_LAT_VEL"
  Switch6/1 -> Bus Creator1/5  "LL_MIN_LANE_WIDTH_ENABLE"
  LL_MIN_LANE_WIDTH_ENABLE=2.5/1 -> Switch6/3
  Data Type Conversion43/1 -> Switch20/1, Switch20/2
  Data Type Conversion38/1 -> Switch18/1, Switch18/2
  LL_MAX_STEER_ANGLE_ENABLE=60/1 -> Switch8/3
  Data Type Conversion40/1 -> Switch13/1, Switch13/2
  LL_LKA_LatestWarnLine_C=-0.5/1 -> Switch20/3
  ICv to v2/1(Out1) -> Bus Creator1/3  "LL_MIN_LKAS_SPEED_ENABLE"
  Data Type Conversion42/1 -> Switch19/1, Switch19/2
  LL_MAX_LANE_WIDTH_ENABLE=5.4/1 -> Switch7/3
  Switch10/1 -> Bus Creator1/9  "LL_MAX_STEER_SPEED_ENABLE"
  Data Type Conversion39/1 -> Switch12/1, Switch12/2

== system LKAS_AutoSave_20200910_1510/LKAS/SignalBusCreator/DTC_Indicator ==
  Bus Creator11 : BusCreator  Inputs=2
  Constant{,2..21} (21 alike) : Constant  Value=0  OutDataTypeStr=uint8
  Mux : Mux  Inputs=16
  Mux1 : Mux  Inputs=5
  bsDTC_Indicator : Outport
  wires:
  Bus Creator11/1 -> bsDTC_Indicator/1  "bsDTC_Indicator"
  Mux/1 -> Bus Creator11/1  "LKAS_BSWDTC_Status"
  Constant/1 -> Mux/1  "CANEve_e_BusOff_PSA1CAN"
  Constant2/1 -> Mux/2  "CANEve_e_BusOff_SensorCAN"
  Constant4/1 -> Mux/4  "CANEve_e_Node_ESC_Validity"
  Constant3/1 -> Mux/3  "CANEve_e_Mute_PSA1CAN"
  Constant7/1 -> Mux/7  "CANEve_e_Node_TCU_Validity"
  Constant8/1 -> Mux/8  "CANEve_e_Node_GW_Validity"
  Constant6/1 -> Mux/6  "CANEve_e_Node_EMS_Validity"
  Constant5/1 -> Mux/5  "CANEve_e_Node_EPS_Validity"
  Constant13/1 -> Mux/13  "Reserved3"
  Constant14/1 -> Mux/14  "Reserved4"
  Constant16/1 -> Mux/16  "Reserved6"
  Constant15/1 -> Mux/15  "Reserved5"
  Constant11/1 -> Mux/11  "Reserved1"
  Constant12/1 -> Mux/12  "Reserved2"
  Constant10/1 -> Mux/10  "CANEve_e_Node_Camera_Validity"
  Constant9/1 -> Mux/9  "CANEve_e_Node_Radar_Validity"
  Constant17/1 -> Mux1/1  "ACC"
  Constant18/1 -> Mux1/2  "AEB"
  Constant19/1 -> Mux1/3  "LKA"
  Constant20/1 -> Mux1/4  "LDW"
  Constant21/1 -> Mux1/5  "TJA"
  Mux1/1 -> Bus Creator11/2  "Indicator_Status"

== system LKAS_AutoSave_20200910_1510/LKAS/SignalBusCreator/Fusion_AdditionalInf ==
  Bus Creator11 : BusCreator  Inputs=10
  Constant{,1..9} (10 alike) : Constant  Value=0  OutDataTypeStr=uint8
  Fusion_AdditionalInf : Outport
  wires:
  Constant1/1 -> Bus Creator11/2  "Radar_State"
  Constant3/1 -> Bus Creator11/4  "fusion_status"
  Constant6/1 -> Bus Creator11/7  "CONSTRUCTION_AREA"
  Constant2/1 -> Bus Creator11/3  "sensor_status"
  Constant4/1 -> Bus Creator11/5  "fusion_time_stamp"
  Constant5/1 -> Bus Creator11/6  "LANE_DETECT_ACTIV"
  Constant/1 -> Bus Creator11/1  "Carema_Status"
  Constant9/1 -> Bus Creator11/10  "SIGN_TSR_Sign_Type"
  Constant7/1 -> Bus Creator11/8  "ROAD_TYPE"
  Constant8/1 -> Bus Creator11/9  "SIGN_ISA_Value"
  Bus Creator11/1 -> Fusion_AdditionalInf/1  "Fusion_AdditionalInf"

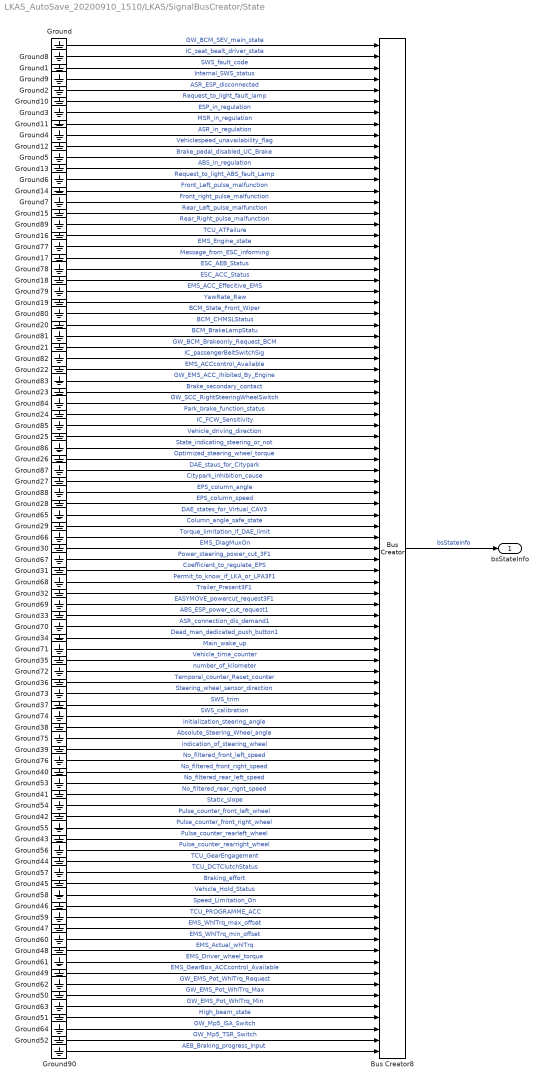
== system LKAS_AutoSave_20200910_1510/LKAS/SignalBusCreator/State ==
  Bus Creator8 : BusCreator  Inputs=91
  Ground{,1..90} (91 alike) : Ground
  bsStateInfo : Outport
  wires:
  Ground14/1 -> Bus Creator8/14  "Front_Left_pulse_malfunction"
  Ground8/1 -> Bus Creator8/2  "IC_seat_bealt_driver_state"
  Ground/1 -> Bus Creator8/1  "GW_BCM_SEV_main_state"
  Ground42/1 -> Bus Creator8/70  "Pulse_counter_front_left_wheel"
  Ground43/1 -> Bus Creator8/72  "Pulse_counter_rearleft_wheel"
  Ground12/1 -> Bus Creator8/10  "Vehiclespeed_unavailability_flag"
  Ground75/1 -> Bus Creator8/63  "Absolute_Steering_Wheel_angle"
  Ground71/1 -> Bus Creator8/55  "Main_wake_up"
  Ground44/1 -> Bus Creator8/74  "TCU_GearEngagement"
  Ground55/1 -> Bus Creator8/71  "Pulse_counter_front_right_wheel"
  Ground7/1 -> Bus Creator8/15  "Front_right_pulse_malfunction"
  Ground28/1 -> Bus Creator8/42  "EPS_column_speed"
  Ground79/1 -> Bus Creator8/23  "EMS_ACC_Effecitive_EMS"
  Ground77/1 -> Bus Creator8/19  "EMS_Engine_state"
  Ground80/1 -> Bus Creator8/25  "BCM_State_Front_Wiper"
  Ground41/1 -> Bus Creator8/68  "No_filtered_rear_rignt_speed"
  Ground67/1 -> Bus Creator8/47  "Power_steering_power_cut_3F1"
  Bus Creator8/1 -> bsStateInfo/1  "bsStateInfo"
  Ground90/1 -> Bus Creator8/91  "AEB_Braking_progress_Input"
  Ground38/1 -> Bus Creator8/62  "Initialization_steering_angle"
  Ground19/1 -> Bus Creator8/24  "YawRate_Raw"
  Ground83/1 -> Bus Creator8/31  "GW_EMS_ACC_Ihibited_By_Engine"
  Ground46/1 -> Bus Creator8/78  "Speed_Limitation_On"
  Ground51/1 -> Bus Creator8/88  "High_beam_state"
  Ground40/1 -> Bus Creator8/66  "No_filtered_front_right_speed"
  Ground3/1 -> Bus Creator8/7  "ESP_in_regulation"
  Ground36/1 -> Bus Creator8/58  "Temporal_counter_Reset_counter"
  Ground11/1 -> Bus Creator8/8  "MSR_in_regulation"
  Ground50/1 -> Bus Creator8/86  "GW_EMS_Pot_WhlTrq_Max"
  Ground10/1 -> Bus Creator8/6  "Request_to_light_fault_lamp"
  Ground13/1 -> Bus Creator8/12  "ABS_in_regulation"
  Ground5/1 -> Bus Creator8/11  "Brake_pedal_disabled_UC_Brake"
  Ground23/1 -> Bus Creator8/32  "Brake_secondary_contact"
  Ground60/1 -> Bus Creator8/81  "EMS_WhlTrq_min_offset"
  Ground15/1 -> Bus Creator8/16  "Rear_Left_pulse_malfunction"
  Ground24/1 -> Bus Creator8/34  "Park_brake_function_status"
  Ground6/1 -> Bus Creator8/13  "Request_to_light_ABS_fault_Lamp"
  Ground66/1 -> Bus Creator8/45  "Torque_limitation_if_DAE_limit"
  Ground72/1 -> Bus Creator8/57  "number_of_kilometer"
  Ground9/1 -> Bus Creator8/4  "Internal_SWS_status"
  Ground31/1 -> Bus Creator8/48  "Coefficient_to_regulate_EPS"
  Ground89/1 -> Bus Creator8/17  "Rear_Right_pulse_malfunction"
  Ground22/1 -> Bus Creator8/30  "EMS_ACCcontrol_Available"
  Ground73/1 -> Bus Creator8/59  "Steering_wheel_sensor_direction"
  Ground52/1 -> Bus Creator8/90  "GW_Mp5_TSR_Switch"
  Ground54/1 -> Bus Creator8/69  "Static_slope"
  Ground63/1 -> Bus Creator8/87  "GW_EMS_Pot_WhlTrq_Min"
  Ground25/1 -> Bus Creator8/36  "Vehicle_driving_direction"
  Ground69/1 -> Bus Creator8/51  "EASYMOVE_powercut_request3F1"
  Ground39/1 -> Bus Creator8/64  "indication_of_steering_wheel"
  Ground20/1 -> Bus Creator8/26  "BCM_CHMSLStatus"
  Ground57/1 -> Bus Creator8/75  "TCU_DCTClutchStatus"
  Ground27/1 -> Bus Creator8/40  "Citypark_inhibition_cause"
  Ground18/1 -> Bus Creator8/22  "ESC_ACC_Status"
  Ground65/1 -> Bus Creator8/43  "DAE_states_for_Virtual_CAV3"
  Ground84/1 -> Bus Creator8/33  "GW_SCC_RightSteeringWheelSwitch"
  Ground26/1 -> Bus Creator8/38  "Optimized_steering_wheel_torque"
  Ground33/1 -> Bus Creator8/52  "ABS_ESP_power_cut_request1"
  Ground17/1 -> Bus Creator8/20  "Message_from_ESC_informing"
  Ground29/1 -> Bus Creator8/44  "Column_angle_safe_state"
  Ground30/1 -> Bus Creator8/46  "EMS_DiagMuxOn"
  Ground68/1 -> Bus Creator8/49  "Permit_to_know_if_LKA_or_LPA3F1"
  Ground70/1 -> Bus Creator8/53  "ASR_connection_dis_demand1"
  Ground74/1 -> Bus Creator8/61  "SWS_calibration"
  Ground4/1 -> Bus Creator8/9  "ASR_in_regulation"
  Ground37/1 -> Bus Creator8/60  "SWS_trim"
  Ground53/1 -> Bus Creator8/67  "No_filtered_rear_left_speed"
  Ground2/1 -> Bus Creator8/5  "ASR_ESP_disconnected"
  Ground56/1 -> Bus Creator8/73  "Pulse_counter_rearright_wheel"
  Ground21/1 -> Bus Creator8/28  "GW_BCM_Brakeonly_Request_BCM"
  Ground59/1 -> Bus Creator8/79  "TCU_PROGRAMME_ACC"
  Ground47/1 -> Bus Creator8/80  "EMS_WhlTrq_max_offset"
  Ground45/1 -> Bus Creator8/76  "Braking_effort"
  Ground48/1 -> Bus Creator8/82  "EMS_Actual_whlTrq"
  Ground49/1 -> Bus Creator8/84  "EMS_GearBox_ACCcontrol_Available"
  Ground87/1 -> Bus Creator8/39  "DAE_staus_for_Citypark"
  Ground86/1 -> Bus Creator8/37  "State_indicating_steering_or_not"
  Ground85/1 -> Bus Creator8/35  "IC_FCW_Sensitivity"
  Ground78/1 -> Bus Creator8/21  "ESC_AEB_Status"
  Ground82/1 -> Bus Creator8/29  "IC_passengerBeltSwitchSig"
  Ground81/1 -> Bus Creator8/27  "BCM_BrakeLampStatu"
  Ground58/1 -> Bus Creator8/77  "Vehicle_Hold_Status"
  Ground64/1 -> Bus Creator8/89  "GW_Mp5_ISA_Switch"
  Ground35/1 -> Bus Creator8/56  "Vehicle_time_counter"
  Ground34/1 -> Bus Creator8/54  "Dead_man_dedicated_push_button1"
  Ground32/1 -> Bus Creator8/50  "Trailer_Present3F1"
  Ground61/1 -> Bus Creator8/83  "EMS_Driver_wheel_torque"
  Ground76/1 -> Bus Creator8/65  "No_filtered_front_left_speed"
  Ground62/1 -> Bus Creator8/85  "GW_EMS_Pot_WhlTrq_Request"
  Ground88/1 -> Bus Creator8/41  "EPS_column_angle"
  Ground16/1 -> Bus Creator8/18  "TCU_ATFailure"
  Ground1/1 -> Bus Creator8/3  "SWS_fault_code"

== system LKAS_AutoSave_20200910_1510/LKAS/LL/Human Machine Interface (HMI)/Subsystem ==
  LDW_STATE : Inport
  EPSInfo : Inport  Port=2
  Abs : Abs
  Bus Selector2 : BusSelector  OutputSignals=EPS_LKA_State,EPS_SW_Trq
  Compare1 : simulink/Logic and Bit Operations/Compare To Constant  relop===  const=3  OutDataTypeStr=boolean
  Compare2 : simulink/Logic and Bit Operations/Compare To Constant  relop===  const=3  OutDataTypeStr=boolean
  Compare3 : simulink/Logic and Bit Operations/Compare To Constant  relop===  const=1  OutDataTypeStr=boolean
  Compare4 : simulink/Logic and Bit Operations/Compare To Constant  relop===  const=3  OutDataTypeStr=boolean
  Compare5 : simulink/Logic and Bit Operations/Compare To Constant  relop===  const=4  OutDataTypeStr=boolean
  Compare6 : simulink/Logic and Bit Operations/Compare To Constant  relop===  const=5  OutDataTypeStr=boolean
  Constant : Constant  Value=0.25  OutDataTypeStr=single
  Constant1 : Constant  Value=0.5  OutDataTypeStr=single
  Count 10s : Subsystem
  Count 15s : Subsystem
  Logical Operator2 : Logic  AllPortsSameDT=off  OutDataTypeStr=boolean
  Logical Operator3 : Logic  Operator=OR  Inputs=5  AllPortsSameDT=off  OutDataTypeStr=boolean
  Relational Operator : RelationalOperator  Operator=<=  OutDataTypeStr=boolean  RndMeth=Nearest
  Switch : Switch  Criteria=u2 > Threshold
  HandsOff10s : Outport
  HandsOff15s : Outport  Port=2
  wires:
  Count 10s/1(Out) -> HandsOff10s/1
  Compare3/1 -> Logical Operator3/5
  Compare2/1 -> Logical Operator3/4
  Bus Selector2/1 -> Compare1/1, Compare3/1, Compare2/1  "<EPS_LKA_State>"
  Constant/1 -> Switch/3
  EPSInfo/1 -> Bus Selector2/1
  Switch/1 -> Relational Operator/2
  Compare1/1 -> Switch/2
  Bus Selector2/2 -> Abs/1  "<EPS_SW_Trq>"
  Logical Operator2/1 -> Count 15s/Enable, Count 10s/Enable
  Logical Operator3/1 -> Logical Operator2/1
  Constant1/1 -> Switch/1
  Relational Operator/1 -> Logical Operator2/2
  Count 15s/1(Out) -> HandsOff15s/1
  LDW_STATE/1 -> Compare4/1, Compare6/1, Compare5/1
  Compare4/1 -> Logical Operator3/3
  Compare5/1 -> Logical Operator3/2
  Compare6/1 -> Logical Operator3/1
  Abs/1 -> Relational Operator/1

== system LKAS_AutoSave_20200910_1510/LKAS/LL/LL Inputs Mapping/bsBCMInfo ==
  bsBCMInfoIn : Inport
  Bus Creator1 : BusCreator  Inputs=3
  Bus Selector1 : BusSelector  OutputSignals=BCM_Double_Light,BCM_Left_Light,BCM_Right_Light
  bsBCMInfoOut : Outport
  wires:
  Bus Selector1/3 -> Bus Creator1/3  "<BCM_Right_Light>"
  Bus Selector1/2 -> Bus Creator1/2  "<BCM_Left_Light>"
  Bus Creator1/1 -> bsBCMInfoOut/1
  Bus Selector1/1 -> Bus Creator1/1  "<BCM_Double_Light>"
  bsBCMInfoIn/1 -> Bus Selector1/1

== system LKAS_AutoSave_20200910_1510/LKAS/LL/LL Inputs Mapping/bsEPSInfo ==
  bsEPSInfoIn : Inport
  Bus Creator4 : BusCreator  Inputs=9
  Bus Selector1 : BusSelector  OutputSignals=EPS_LKA_State,EPS_SW_Trq,EPS_Error_State,EPS_Trq_State,SAS_Clb_State,SAS_Trim_State,EPS_TrqLim_State,EPS_LKA_Current,EPS_SWHold_State
  bsEPSInfoOut : Outport
  wires:
  Bus Selector1/9 -> Bus Creator4/9  "<EPS_SWHold_State>"
  Bus Selector1/8 -> Bus Creator4/8  "<EPS_LKA_Current>"
  Bus Selector1/7 -> Bus Creator4/7  "<EPS_TrqLim_State>"
  Bus Selector1/6 -> Bus Creator4/6  "<SAS_Trim_State>"
  Bus Selector1/5 -> Bus Creator4/5  "<SAS_Clb_State>"
  Bus Selector1/4 -> Bus Creator4/4  "<EPS_Trq_State>"
  Bus Selector1/3 -> Bus Creator4/3  "<EPS_Error_State>"
  Bus Creator4/1 -> bsEPSInfoOut/1
  Bus Selector1/1 -> Bus Creator4/1  "<EPS_LKA_State>"
  Bus Selector1/2 -> Bus Creator4/2  "<EPS_SW_Trq>"
  bsEPSInfoIn/1 -> Bus Selector1/1

== system LKAS_AutoSave_20200910_1510/LKAS/LL/LL Inputs Mapping/bsLaneInfo ==
  bsLaneInfoIn : Inport
  Bus Creator : BusCreator  Inputs=7
  Bus Selector1 : BusSelector  OutputSignals=bsFusLaneInfo,bsFusL0Info,bsFusR0Info,bsFusL1Info,bsFusR1Info,bsOriLaneInfo,bsOriL0Info,bsOriR0Info,bsOriL1Info,bsOriR1Info,Fusion_AdditionalInf
  LaneSelect : Subsystem
  "LanesReconstruct " : Subsystem
  bsLaneInfoOut : Outport
  wires:
  Bus Selector1/1 -> Bus Creator/1  "<bsFusLaneInfo>"
  Bus Selector1/6 -> Bus Creator/6  "<bsOriLaneInfo>"
  Bus Creator/1 -> bsLaneInfoOut/1
  Bus Selector1/10 -> LaneSelect/8(bsOriR1Info)  "<bsOriR1Info>"
  Bus Selector1/9 -> LaneSelect/7(bsOriL1Info)  "<bsOriL1Info>"
  Bus Selector1/8 -> LaneSelect/6(bsOriR0Info)  "<bsOriR0Info>"
  Bus Selector1/7 -> LaneSelect/5(bsOriL0Info)  "<bsOriL0Info>"
  Bus Selector1/5 -> LaneSelect/4(bsFusR1Info)  "<bsFusR1Info>"
  Bus Selector1/4 -> LaneSelect/3(bsFusL1Info)  "<bsFusL1Info>"
  Bus Selector1/3 -> LaneSelect/2(bsFusR0Info)  "<bsFusR0Info>"
  Bus Selector1/2 -> LaneSelect/1(bsFusL0Info)  "<bsFusL0Info>"
  LaneSelect/4(bsR1Info) -> "LanesReconstruct "/4(bsR1Info)
  LaneSelect/3(bsL1Info) -> "LanesReconstruct "/3(bsL1Info)
  LaneSelect/2(bsR0Info) -> "LanesReconstruct "/2(bsR0Info)
  LaneSelect/1(bsL0Info) -> "LanesReconstruct "/1(bsL0Info)
  "LanesReconstruct "/4(bsR1InfoR) -> Bus Creator/5  "bsR1Info"
  "LanesReconstruct "/3(bsL1InfoR) -> Bus Creator/4  "bsL1Info"
  "LanesReconstruct "/2(bsR0InfoR) -> Bus Creator/3  "bsR0Info"
  "LanesReconstruct "/1(bsL0InfoR) -> Bus Creator/2  "bsL0Info"
  Bus Selector1/11 -> Bus Creator/7  "<Fusion_AdditionalInf>"
  bsLaneInfoIn/1 -> Bus Selector1/1

== system LKAS_AutoSave_20200910_1510/LKAS/LL/LL Inputs Mapping/bsMP5Info ==
  bsMP5InfoIn : Inport
  Bus Creator4 : BusCreator  Inputs=3
  Bus Selector1 : BusSelector  OutputSignals=LKA_Main_Switch,LKA_Mode,LDW_Warn_Mode
  bsMP5InfoOut : Outport
  wires:
  Bus Selector1/3 -> Bus Creator4/3  "<LDW_Warn_Mode>"
  bsMP5InfoIn/1 -> Bus Selector1/1
  Bus Creator4/1 -> bsMP5InfoOut/1
  Bus Selector1/2 -> Bus Creator4/2  "<LKA_Mode>"
  Bus Selector1/1 -> Bus Creator4/1  "<LKA_Main_Switch>"

== system LKAS_AutoSave_20200910_1510/LKAS/LL/LL Inputs Mapping/bsPTState ==
  bsPTStateIn : Inport
  Bus Creator3 : BusCreator  Inputs=2
  Bus Selector1 : BusSelector  OutputSignals=AccPedal_Pos,TCU_ActualGear
  bsPTStateOut : Outport
  wires:
  Bus Creator3/1 -> bsPTStateOut/1
  Bus Selector1/1 -> Bus Creator3/1  "<AccPedal_Pos>"
  bsPTStateIn/1 -> Bus Selector1/1
  Bus Selector1/2 -> Bus Creator3/2  "<TCU_ActualGear>"

== system LKAS_AutoSave_20200910_1510/LKAS/LL/LL Inputs Mapping/bsSWAInfo ==
  bsSWAInfoIn : Inport
  Bus Creator : BusCreator  Inputs=4
  Bus Selector1 : BusSelector  OutputSignals=SW_Angle,SW_Angle_Speed,SWS_Fault_Code,SAS_In_Status
  bsSWAInfoOut : Outport
  wires:
  Bus Creator/1 -> bsSWAInfoOut/1
  Bus Selector1/4 -> Bus Creator/4  "<SAS_In_Status>"
  Bus Selector1/3 -> Bus Creator/3  "<SWS_Fault_Code>"
  Bus Selector1/2 -> Bus Creator/2  "<SW_Angle_Speed>"
  Bus Selector1/1 -> Bus Creator/1  "<SW_Angle>"
  bsSWAInfoIn/1 -> Bus Selector1/1
